simulink model "PMSM_U_F_PWM"  (R2020a)
settings: Solver=ode3  StartTime=0.0  StopTime=0.5  FixedStep=1e-5  RelTol=1e-3  EnableMultiTasking=on
model workspace (MAT data in the model file):
  B = 2.3e-05
  J = 6.5e-05
  KC = 0.04
  KV = 0.021
  L = 0.00021
  PP = 3
  Power_Supply_V = 18
  R = 0.215
  RLoad = 10
  T_FST_LP = 0.00012
undefined symbols (not defined in the file): sigbuilder_block
libraries: ammclib_bam x3, simulink x1
settings Model: Creator=admin_aboyer  LastModifiedBy=bourlot
settings DataIOCC: ExternalInput=off  InitialState=off  SaveOutput=off  SignalLogging=off  SaveTime=off  ReturnWorkspaceOutputs=off
settings OptimizationCC: BlockReduction=off  DefaultParameterBehavior=Inlined  LifeSpan=1  EfficientTunableParamExpr=on
settings DebuggingCC: InheritedTsInSrcMsg=none  MultiTaskDSMMsg=none  MultiTaskRateTransMsg=warning  SingleTaskRateTransMsg=warning  UnconnectedInputMsg=error  UnconnectedOutputMsg=error  UnconnectedLineMsg=error  UnknownTsInhSupMsg=error  SFUnexpectedBacktrackingDiag=warning  SFNoUnconditionalDefaultTransitionDiag=warning  ArithmeticOperatorsInVariantConditions=warning
settings HardwareCC: ProdBitPerPointer=32  ProdBitPerSizeT=32  ProdBitPerPtrDiffT=32  ProdLargestAtomicInteger=Long  ProdLargestAtomicFloat=Double  ProdEndianess=BigEndian  ProdWordSize=32  ProdHWDeviceType=Motorola PowerPC
settings SFSimCC: SimUseLocalCustomCode=off  MATLABDynamicMemAlloc=off  CustomCodeUndefinedFunction=UseInterfaceOnly
settings RTWCC: Description=Model Based Design Toolbox MPC574xP Code Generation Target  SystemTargetFile=mbd_pnt.tlc  MakeCommand=mbd_pnt_make_rtw COPY_MDLREF_INCLUDES=0  TemplateMakefile=mbd_pnt.tmf  GenerateReport=on  RTWUseLocalCustomCode=off  IncludeHyperlinkInReport=on  LaunchReport=on  GenerateTraceInfo=on  GenerateTraceReport=on  GenerateTraceReportSl=on  GenerateTraceReportSf=on  GenerateTraceReportEml=on
settings CodeAppCC: ForceParamTrailComments=on  IgnoreCustomStorageClasses=off  OperatorAnnotations=on  SimulinkDataObjDesc=on  SFDataObjDesc=on  MATLABFcnDesc=on  InsertBlockDesc=on  StateflowObjectComments=on  MATLABSourceComments=on
settings STFCustomTargetCC: GenerateSampleERTMain=on  CombineOutputUpdateFcns=on  SuppressErrorStatus=on  ERTCustomFileBanners=on  SupportContinuousTime=off  SupportNonInlinedSFcns=off  RemoveResetFunc=on  MATLABClassNameForMDSCustomization=Simulink.SoftwareTarget.ERTCustomization  SystemTargetFile=mbd_pnt.tlc
settings ERTTargetCC: MultiwordLength=2048  GenerateSampleERTMain=on  ParMdlRefBuildCompliant=off  CompOptLevelCompliant=off  ConcurrentExecutionCompliant=off  SuppressErrorStatus=on  ModelStepFunctionPrototypeControlCompliant=off  CPPClassGenCompliant=off  UseToolchainInfoCompliant=off  InlinedParameterPlacement=NonHierarchical  ERTCustomFileTemplate=example_file_process.tlc
settings ConfigComp: CovMetricSettings=dw  CovHtmlReporting=on  CovSaveCumulativeToWorkspaceVar=on  CovSaveSingleToWorkspaceVar=on  CovExternalEMLEnable=off

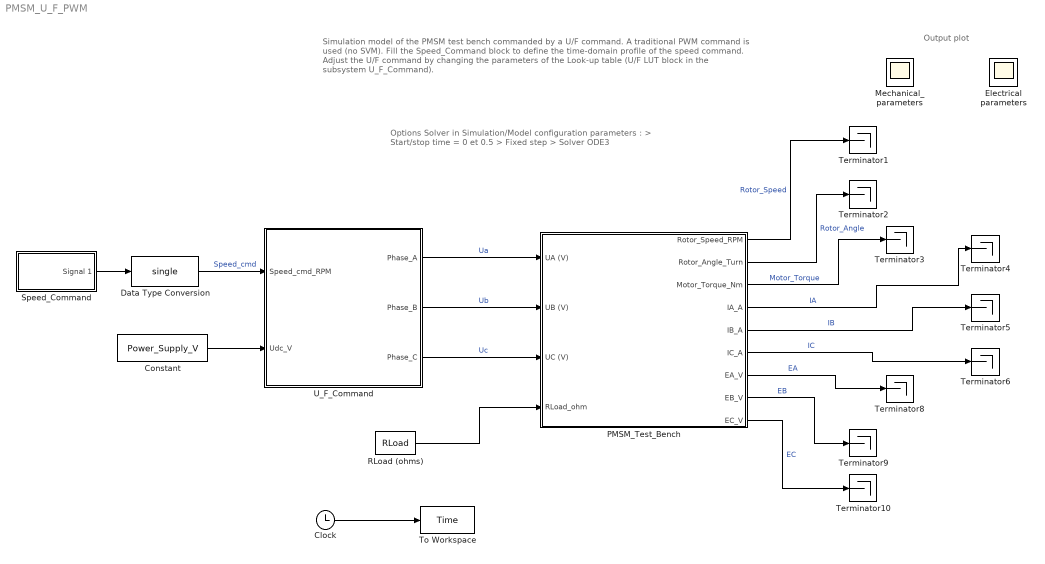
== system PMSM_U_F_PWM ==
  note: Output plot
  note: Options Solver in Simulation/Model configuration parameters :
      | >  Start/stop time = 0 et 0.5
      | >  Fixed step
      | >  Solver ODE3
  note: Simulation model of the PMSM test bench commanded by a U/F command.
      | A traditional PWM command is used (no SVM).
      | Fill the Speed_Command block to define the time-domain profile of the speed command.
      | Adjust the U/F command by changing the parameters of the Look-up table (U/F LUT
      | block in the subsystem U_F_Command).
  Clock : Clock
  Constant : Constant  Value=Power_Supply_V  OutDataTypeStr=single
  Data Type Conversion : DataTypeConversion  OutDataTypeStr=single
  Electrical parameters : Scope
      settings: Floating=on
  Mechanical_parameters : Scope
      settings: Floating=on
  PMSM_Test_Bench : Subsystem
  RLoad (ohms) : Constant  Value=RLoad
  Speed_Command : Subsystem  Tag=STV Subsys  LoadFcn=sigbuilder_block('load');  StartFcn=sigbuilder_block('start');  StopFcn=sigbuilder_block('stop');  ClipboardFcn=sigbuilder_block('clipboard');  mask(Sigbuilder block){tuvar=[0:10]}
      mask help: Simulink:masks:SigbuilderBlock_MD
      mask init:
      | if ~strcmp(get_param(bdroot(gcbh),'SimulationStatus'),'stopped') tuvar = sigbuilder_block('maskInit'); end
      settings: CopyFcn=sigbuilder_block('copy');  DeleteFcn=sigbuilder_block('delete');  ModelCloseFcn=sigbuilder_block('modelClose');  PreSaveFcn=sigbuilder_block('preSave');  PauseFcn=sigbuilder_block('pause');  ContinueFcn=sigbuilder_block('continue');  NameChangeFcn=sigbuilder_block('namechange');  OpenFcn=sigbuilder_block('open',[437.25 153.75 550.5 359.25 ]);  CloseFcn=sigbuilder_block('close');
      mask Display: plot(0, 0, 100, 100,[2, 2, 32, 32, 2], [68, 8, 8, 68, 68],[32, 2], [38, 38], [32, 19, 2],[53, 60, 44], [32, 17, 17, 2],[16, 16, 31, 31]);txt = getActiveGroup(gcbh);text(2, 100, txt,'verticalAlignment', 'top');
  Terminator{1..6,8..10} (9 alike) : Terminator
  To Workspace : ToWorkspace  VariableName=Time  SampleTime=-1
  U_F_Command : Subsystem
  wires:
  Clock/1 -> To Workspace/1
  U_F_Command/1(Phase_A) -> PMSM_Test_Bench/1(UA (V))  "Ua"
  U_F_Command/2(Phase_B) -> PMSM_Test_Bench/2(UB (V))  "Ub"
  U_F_Command/3(Phase_C) -> PMSM_Test_Bench/3(UC (V))  "Uc"
  PMSM_Test_Bench/1(Rotor_Speed_RPM) -> Terminator1/1  "Rotor_Speed"
  PMSM_Test_Bench/2(Rotor_Angle_Turn) -> Terminator2/1  "Rotor_Angle"
  PMSM_Test_Bench/3(Motor_Torque_Nm) -> Terminator3/1  "Motor_Torque"
  PMSM_Test_Bench/4(IA_A) -> Terminator4/1  "IA"
  PMSM_Test_Bench/5(IB_A) -> Terminator5/1  "IB"
  PMSM_Test_Bench/6(IC_A) -> Terminator6/1  "IC"
  PMSM_Test_Bench/7(EA_V) -> Terminator8/1  "EA"
  PMSM_Test_Bench/8(EB_V) -> Terminator9/1  "EB"
  PMSM_Test_Bench/9(EC_V) -> Terminator10/1  "EC"
  RLoad (ohms)/1 -> PMSM_Test_Bench/4(RLoad_ohm)
  Speed_Command/1(Signal 1) -> Data Type Conversion/1
  Data Type Conversion/1 -> U_F_Command/1(Speed_cmd_RPM)  "Speed_cmd"
  Constant/1 -> U_F_Command/2(Udc_V)

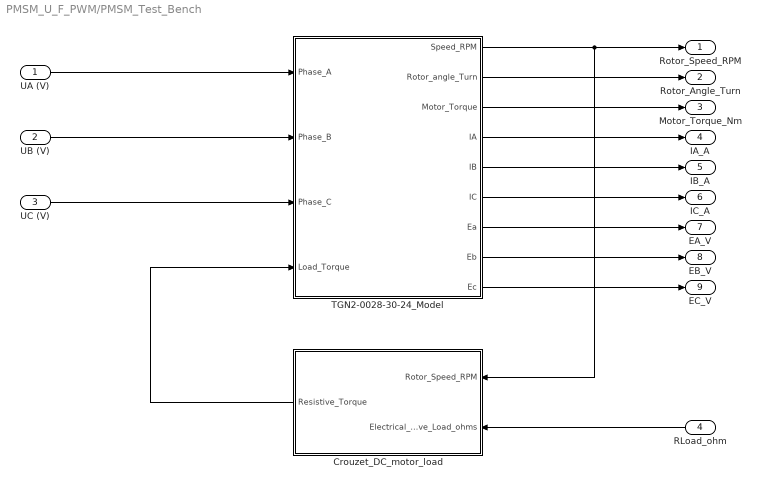
== system PMSM_U_F_PWM/PMSM_Test_Bench ==
  UA (V) : Inport
  UB (V) : Inport  Port=2
  UC (V) : Inport  Port=3
  RLoad_ohm : Inport  Port=4
  Crouzet_DC_motor_load : Subsystem
  TGN2-0028-30-24_Model : Subsystem
      mask Display: image('C:\WORKSPACE_MATLAB\PMSM_Workshop\M5\img\PMSM.PNG');
  Rotor_Speed_RPM : Outport
  Rotor_Angle_Turn : Outport  Port=2
  Motor_Torque_Nm : Outport  Port=3
  IA_A : Outport  Port=4
  IB_A : Outport  Port=5
  IC_A : Outport  Port=6
  EA_V : Outport  Port=7
  EB_V : Outport  Port=8
  EC_V : Outport  Port=9
  wires:
  Crouzet_DC_motor_load/1(Resistive_Torque) -> TGN2-0028-30-24_Model/4(Load_Torque)
  TGN2-0028-30-24_Model/1(Speed_RPM) -> Rotor_Speed_RPM/1, Crouzet_DC_motor_load/1(Rotor_Speed_RPM)
  UA (V)/1 -> TGN2-0028-30-24_Model/1(Phase_A)
  UB (V)/1 -> TGN2-0028-30-24_Model/2(Phase_B)
  UC (V)/1 -> TGN2-0028-30-24_Model/3(Phase_C)
  TGN2-0028-30-24_Model/2(Rotor_angle_Turn) -> Rotor_Angle_Turn/1
  TGN2-0028-30-24_Model/3(Motor_Torque) -> Motor_Torque_Nm/1
  TGN2-0028-30-24_Model/4(IA) -> IA_A/1
  TGN2-0028-30-24_Model/5(IB) -> IB_A/1
  TGN2-0028-30-24_Model/6(IC) -> IC_A/1
  TGN2-0028-30-24_Model/7(Ea) -> EA_V/1
  TGN2-0028-30-24_Model/8(Eb) -> EB_V/1
  TGN2-0028-30-24_Model/9(Ec) -> EC_V/1
  RLoad_ohm/1 -> Crouzet_DC_motor_load/2(Electrical_resistive_Load_ohms)

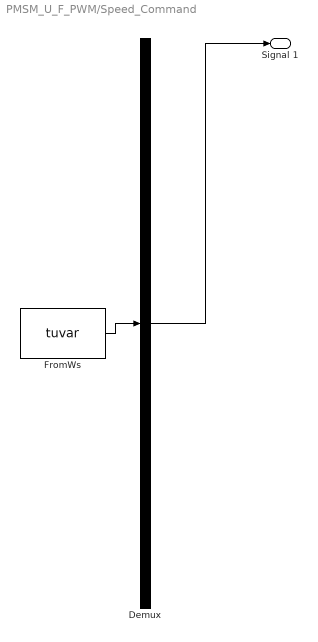
== system PMSM_U_F_PWM/Speed_Command ==
  Demux : Demux  Tag=STV Demux  Outputs=1
      settings: DisplayOption=none
  FromWs : FromWorkspace  Tag=STV FromWs  VariableName=tuvar
      SigBuilderData=|
      | common.afterFinalStr = 'Extrapolate'
      | common.sampleTime = 0
      | dataSet.timeRange = [0 10]
      | dataSet.name = 'Group 1'
      | sbobj.Groups.Name = 'Group 1'
      | sbobj.Groups.Signals.Name = 'Signal 1'
      | sbobj.Groups.Signals.XData = [0 0.2 6 10]
      | sbobj.Groups.Signals.YData = [0 1000 1000 0]
  Signal 1 : Outport  Tag=STV Outport
  wires:
  Demux/1 -> Signal 1/1
  FromWs/1 -> Demux/1

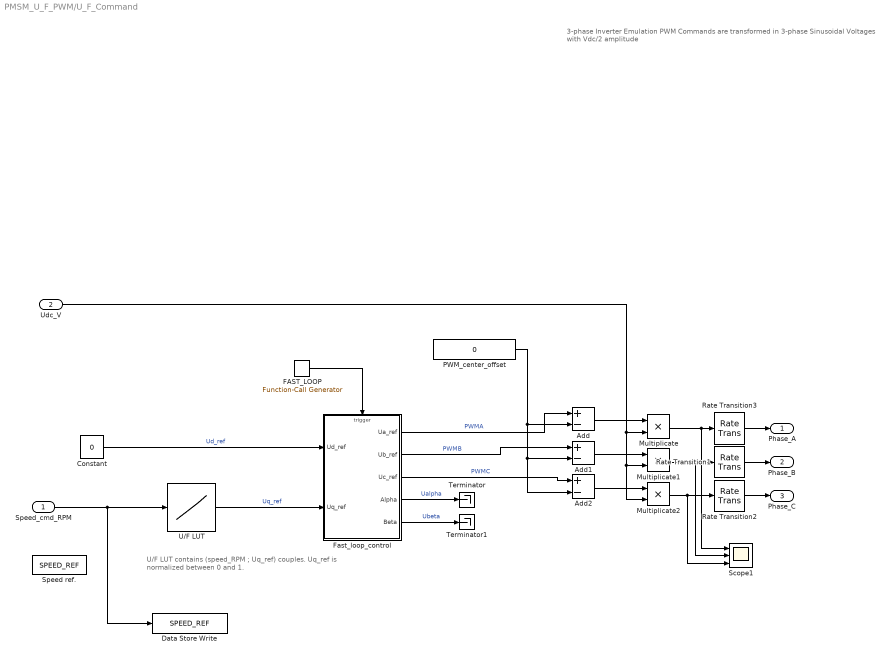
== system PMSM_U_F_PWM/U_F_Command ==
  note: U/F LUT contains (speed_RPM ; Uq_ref) couples. Uq_ref
      | is normalized between 0 and 1.
  note: 3-phase Inverter Emulation
      |
      | PWM Commands are transformed in 3-phase Sinusoidal Voltages with Vdc/2 amplitude
  Speed_cmd_RPM : Inport  OutDataTypeStr=single
  Udc_V : Inport  Port=2
  Add : Sum  Inputs=+-  OutDataTypeStr=single
  Add1 : Sum  Inputs=+-  OutDataTypeStr=single
  Add2 : Sum  Inputs=+-  OutDataTypeStr=single
  Constant : Constant  Value=0  OutDataTypeStr=single
  Data Store Write : DataStoreWrite  DataStoreName=SPEED_REF
  FAST_LOOP : simulink/Ports & Subsystems/Function-Call Generator  sample_time=T_FST_LP  numberOfIterations=1
  Fast_loop_control : Subsystem
  Multiplicate : Product  Inputs=**  OutDataTypeStr=single
  Multiplicate1 : Product  Inputs=**  OutDataTypeStr=single
  Multiplicate2 : Product  Inputs=**  OutDataTypeStr=single
  PWM_center_offset : Constant  Value=0  OutDataTypeStr=single
  Rate Transition1 : RateTransition
  Rate Transition2 : RateTransition
  Rate Transition3 : RateTransition
  Scope1 : Scope  NumInputPorts=3
  Speed ref. : DataStoreMemory  DataStoreName=SPEED_REF  ReadBeforeWriteMsg=warning  WriteAfterWriteMsg=warning  WriteAfterReadMsg=warning  ShowAdditionalParam=off  OutDataTypeStr=single
  Terminator : Terminator
  Terminator1 : Terminator
  U/F LUT : Lookup_n-D  NumberOfTableDimensions=1  BreakpointsForDimension1=[0,500,1000,2571,3000]  Table=[0.194,0.194,0.39,1,1]  InternalRulePriority=Speed  RndMeth=Simplest  InputSameDT=on
  Phase_A : Outport
  Phase_B : Outport  Port=2
  Phase_C : Outport  Port=3
  wires:
  FAST_LOOP/1 -> Fast_loop_control/Trigger
  Fast_loop_control/1(Ua_ref) -> Add/1  "PWMA"
  Fast_loop_control/2(Ub_ref) -> Add1/1  "PWMB"
  Fast_loop_control/3(Uc_ref) -> Add2/1  "PWMC"
  Speed_cmd_RPM/1 -> U/F LUT/1, Data Store Write/1
  Constant/1 -> Fast_loop_control/1(Ud_ref)  "Ud_ref"
  Fast_loop_control/4(Alpha) -> Terminator/1  "Ualpha"
  Fast_loop_control/5(Beta) -> Terminator1/1  "Ubeta"
  U/F LUT/1 -> Fast_loop_control/2(Uq_ref)  "Uq_ref"
  PWM_center_offset/1 -> Add/2, Add1/2, Add2/2
  Add/1 -> Multiplicate/1
  Multiplicate/1 -> Scope1/1, Rate Transition3/1
  Add1/1 -> Multiplicate1/1
  Add2/1 -> Multiplicate2/1
  Multiplicate1/1 -> Scope1/2, Rate Transition1/1
  Multiplicate2/1 -> Scope1/3, Rate Transition2/1
  Rate Transition3/1 -> Phase_A/1
  Rate Transition1/1 -> Phase_B/1
  Rate Transition2/1 -> Phase_C/1
  Udc_V/1 -> Multiplicate2/2, Multiplicate1/2, Multiplicate/2

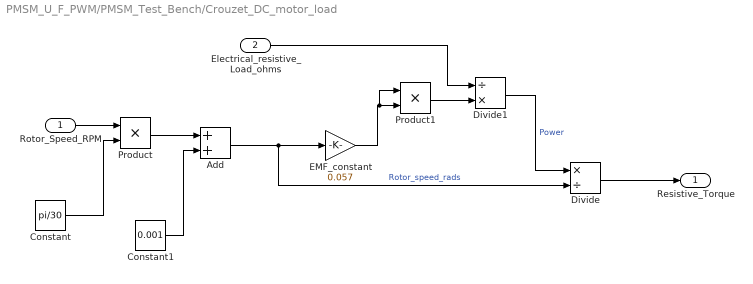
== system PMSM_U_F_PWM/PMSM_Test_Bench/Crouzet_DC_motor_load ==
  Rotor_Speed_RPM : Inport
  Electrical_resistive_Load_ohms : Inport  Port=2
  Add : Sum
  Constant : Constant  Value=pi/30
  Constant1 : Constant  Value=0.001
  Divide : Product  Inputs=*/
  Divide1 : Product  Inputs=/*
  EMF_constant : Gain  Gain=0.057
  Product : Product
  Product1 : Product
  Resistive_Torque : Outport
  wires:
  Rotor_Speed_RPM/1 -> Product/1
  Constant/1 -> Product/2
  Product/1 -> Add/1
  Constant1/1 -> Add/2
  Add/1 -> Divide/2, EMF_constant/1  "Rotor_speed_rads"
  EMF_constant/1 -> Product1/1, Product1/2
  Product1/1 -> Divide1/2
  Divide1/1 -> Divide/1  "Power"
  Divide/1 -> Resistive_Torque/1
  Electrical_resistive_Load_ohms/1 -> Divide1/1

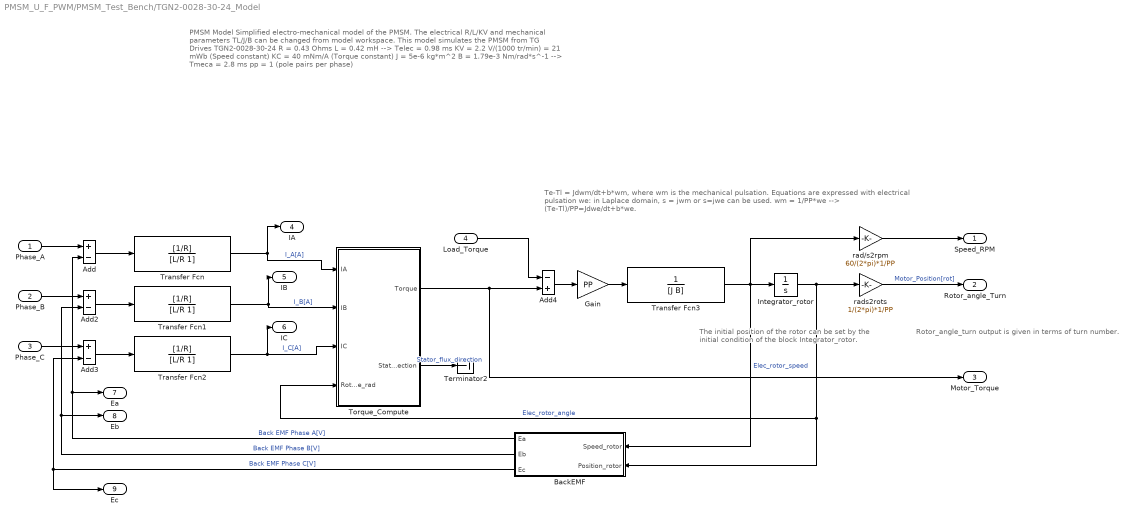
== system PMSM_U_F_PWM/PMSM_Test_Bench/TGN2-0028-30-24_Model ==
  note: The initial position of the rotor can be set by the
      | initial condition of the block Integrator_rotor.
  note: Te-Tl = Jdwm/dt+b*wm, where wm is the mechanical pulsation.
      | Equations are expressed with electrical pulsation we: in Laplace domain, s = jwm or s=jwe can be used.
      | wm = 1/PP*we --> (Te-Tl)/PP=Jdwe/dt+b*we.
  note: PMSM Model
      |
      | Simplified electro-mechanical model of the PMSM. The electrical R/L/KV and mechanical parameters TL/J/B can be changed from model workspace.
      |
      | This model simulates the PMSM from TG Drives TGN2-0028-30-24
      | R = 0.43 Ohms
      | L = 0.42 mH --> Telec = 0.98 ms
      | KV = 2.2 V/(1000 tr/min) = 21 mWb (Speed constant)
      | KC = 40 mNm/A (Torque constant)
      | J = 5e-6 kg*m^2
      | B = 1.79e-3 Nm/rad*s^-1 --> Tmeca = 2.8 ms
      | pp = 1 (pole pairs per phase)
  note: Rotor_angle_turn output is given in terms of turn number.
  Phase_A : Inport
  Phase_B : Inport  Port=2
  Phase_C : Inport  Port=3
  Load_Torque : Inport  Port=4
  Add : Sum  Inputs=+-
  Add2 : Sum  Inputs=+-
  Add3 : Sum  Inputs=+-
  Add4 : Sum  Inputs=-+
  BackEMF : Subsystem
  Gain : Gain  Gain=PP
  Integrator_rotor : Integrator  InitialCondition=-pi/2
  Terminator2 : Terminator
  Torque_Compute : Subsystem
  Transfer Fcn : TransferFcn  Numerator=[1/R]  Denominator=[L/R 1]
  Transfer Fcn1 : TransferFcn  Numerator=[1/R]  Denominator=[L/R 1]
  Transfer Fcn2 : TransferFcn  Numerator=[1/R]  Denominator=[L/R 1]
  Transfer Fcn3 : TransferFcn  Denominator=[J B]
  rad/s2rpm : Gain  Gain=60/(2*pi)*1/PP
  rads2rots : Gain  Gain=1/(2*pi)*1/PP
  Speed_RPM : Outport
  Rotor_angle_Turn : Outport  Port=2
  Motor_Torque : Outport  Port=3
  IA : Outport  Port=4
  IB : Outport  Port=5
  IC : Outport  Port=6
  Ea : Outport  Port=7
  Eb : Outport  Port=8
  Ec : Outport  Port=9
  wires:
  Add/1 -> Transfer Fcn/1
  Phase_A/1 -> Add/1
  Transfer Fcn/1 -> Torque_Compute/1(IA), IA/1  "I_A[A]"
  Transfer Fcn1/1 -> IB/1, Torque_Compute/2(IB)  "I_B[A]"
  Add2/1 -> Transfer Fcn1/1
  Add3/1 -> Transfer Fcn2/1
  Transfer Fcn2/1 -> IC/1, Torque_Compute/3(IC)  "I_C[A]"
  Phase_B/1 -> Add2/1
  Phase_C/1 -> Add3/1
  Load_Torque/1 -> Add4/1
  Add4/1 -> Gain/1
  Gain/1 -> Transfer Fcn3/1
  Transfer Fcn3/1 -> BackEMF/1(Speed_rotor), Integrator_rotor/1, rad/s2rpm/1  "Elec_rotor_speed"
  Torque_Compute/1(Torque) -> Motor_Torque/1, Add4/2
  BackEMF/3(Ec) -> Add3/2, Ec/1  "Back EMF Phase C[V]"
  BackEMF/1(Ea) -> Ea/1, Add/2  "Back EMF Phase A[V]"
  BackEMF/2(Eb) -> Eb/1, Add2/2  "Back EMF Phase B[V]"
  rad/s2rpm/1 -> Speed_RPM/1
  Integrator_rotor/1 -> Torque_Compute/4(Rotor_angle_rad), BackEMF/2(Position_rotor), rads2rots/1  "Elec_rotor_angle"
  rads2rots/1 -> Rotor_angle_Turn/1  "Motor_Position[rot]"
  Torque_Compute/2(Stator_Flux_Direction) -> Terminator2/1  "Stator_flux_direction"

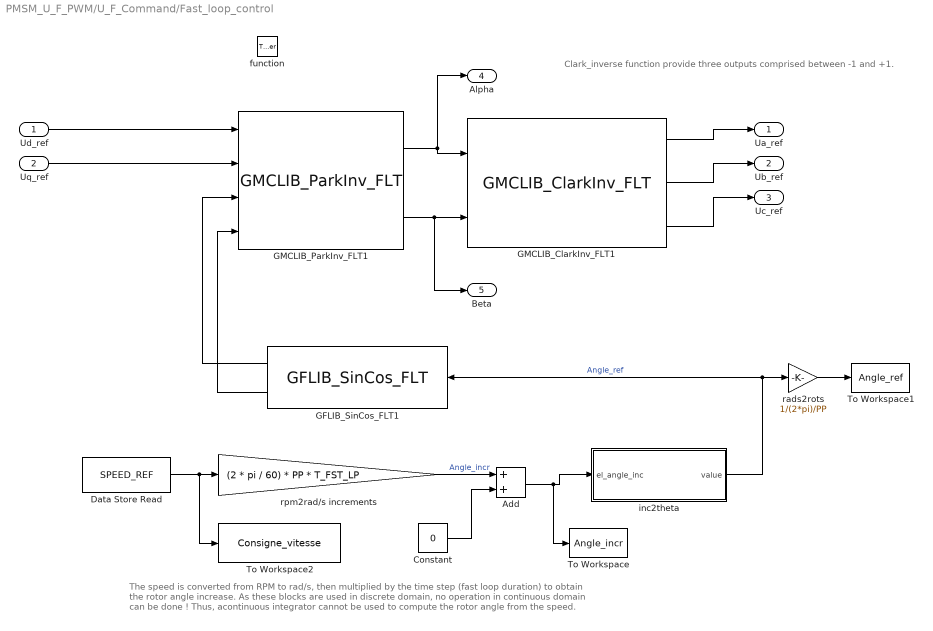
== system PMSM_U_F_PWM/U_F_Command/Fast_loop_control ==
  note: Clark_inverse function provide three outputs comprised between -1 and +1.
  note: The speed is converted from RPM to rad/s, then multiplied by the time step (fast loop duration) to obtain the rotor angle increase.
      | As these blocks are used in discrete domain, no operation in continuous domain can be done ! Thus, acontinuous integrator
      | cannot be used to compute the rotor angle from the speed.
  Ud_ref : Inport
  Uq_ref : Inport  Port=2
  function : TriggerPort  TriggerType=function-call  VariantControl=Variant
  Add : Sum
  Constant : Constant  Value=0  OutDataTypeStr=single
  Data Store Read : DataStoreRead  DataStoreName=SPEED_REF
  GFLIB_SinCos_FLT1 : ammclib_bam/GFLIB/FLT/GFLIB_SinCos_FLT
  GMCLIB_ClarkInv_FLT1 : ammclib_bam/GMCLIB/FLT/GMCLIB_ClarkInv_FLT
  GMCLIB_ParkInv_FLT1 : ammclib_bam/GMCLIB/FLT/GMCLIB_ParkInv_FLT
  To Workspace : ToWorkspace  VariableName=Angle_incr  SampleTime=-1
  To Workspace1 : ToWorkspace  VariableName=Angle_ref  SampleTime=-1
  To Workspace2 : ToWorkspace  VariableName=Consigne_vitesse  SampleTime=-1
  inc2theta : Stateflow chart  TreatAsAtomicUnit=on
      settings: RTWSystemCode=Nonreusable function  RTWFcnNameOpts=Use subsystem name
  rads2rots : Gain  Gain=1/(2*pi)/PP
  rpm2rad/s increments : Gain  Gain=(2 * pi / 60) * PP * T_FST_LP  OutDataTypeStr=single
  Ua_ref : Outport
  Ub_ref : Outport  Port=2
  Uc_ref : Outport  Port=3
  Alpha : Outport  Port=4
  Beta : Outport  Port=5
  wires:
  Data Store Read/1 -> To Workspace2/1, rpm2rad/s increments/1
  inc2theta/1(value) -> GFLIB_SinCos_FLT1/1, rads2rots/1  "Angle_ref"
  GFLIB_SinCos_FLT1/1 -> GMCLIB_ParkInv_FLT1/3
  GMCLIB_ParkInv_FLT1/1 -> GMCLIB_ClarkInv_FLT1/1, Alpha/1
  GMCLIB_ParkInv_FLT1/2 -> GMCLIB_ClarkInv_FLT1/2, Beta/1
  GMCLIB_ClarkInv_FLT1/3 -> Uc_ref/1
  GMCLIB_ClarkInv_FLT1/2 -> Ub_ref/1
  GMCLIB_ClarkInv_FLT1/1 -> Ua_ref/1
  rads2rots/1 -> To Workspace1/1
  rpm2rad/s increments/1 -> Add/1  "Angle_incr"
  Add/1 -> To Workspace/1, inc2theta/1(el_angle_inc)
  Constant/1 -> Add/2
  Uq_ref/1 -> GMCLIB_ParkInv_FLT1/2
  Ud_ref/1 -> GMCLIB_ParkInv_FLT1/1
  GFLIB_SinCos_FLT1/2 -> GMCLIB_ParkInv_FLT1/4

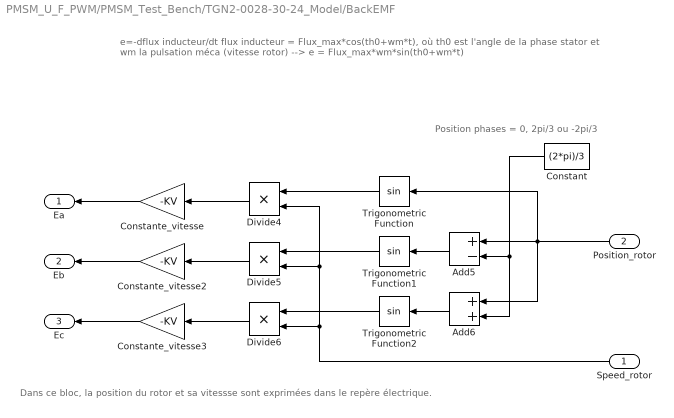
== system PMSM_U_F_PWM/PMSM_Test_Bench/TGN2-0028-30-24_Model/BackEMF ==
  note: Dans ce bloc, la position du rotor et sa vitessse sont exprimées dans le repère électrique.
  note: e=-dflux inducteur/dt
      | flux inducteur = Flux_max*cos(th0+wm*t), où th0 est l'angle de la phase stator et wm la pulsation méca (vitesse rotor)
      | --> e = Flux_max*wm*sin(th0+wm*t)
  note: Position phases = 0, 2pi/3 ou -2pi/3
  Speed_rotor : Inport
  Position_rotor : Inport  Port=2
  Add5 : Sum  Inputs=+-
  Add6 : Sum
  Constant : Constant  Value=(2*pi)/3
  Constante_vitesse : Gain  Gain=-KV
  Constante_vitesse2 : Gain  Gain=-KV
  Constante_vitesse3 : Gain  Gain=-KV
  Divide4 : Product  Inputs=**
  Divide5 : Product  Inputs=**
  Divide6 : Product  Inputs=**
  Trigonometric Function : Trigonometry
  Trigonometric Function1 : Trigonometry
  Trigonometric Function2 : Trigonometry
  Ea : Outport
  Eb : Outport  Port=2
  Ec : Outport  Port=3
  wires:
  Divide4/1 -> Constante_vitesse/1
  Divide6/1 -> Constante_vitesse3/1
  Trigonometric Function2/1 -> Divide6/1
  Constante_vitesse3/1 -> Ec/1
  Speed_rotor/1 -> Divide4/2, Divide5/2, Divide6/2
  Constante_vitesse2/1 -> Eb/1
  Divide5/1 -> Constante_vitesse2/1
  Constant/1 -> Add6/2, Add5/2
  Add6/1 -> Trigonometric Function2/1
  Trigonometric Function/1 -> Divide4/1
  Add5/1 -> Trigonometric Function1/1
  Constante_vitesse/1 -> Ea/1
  Trigonometric Function1/1 -> Divide5/1
  Position_rotor/1 -> Add5/1, Trigonometric Function/1, Add6/1

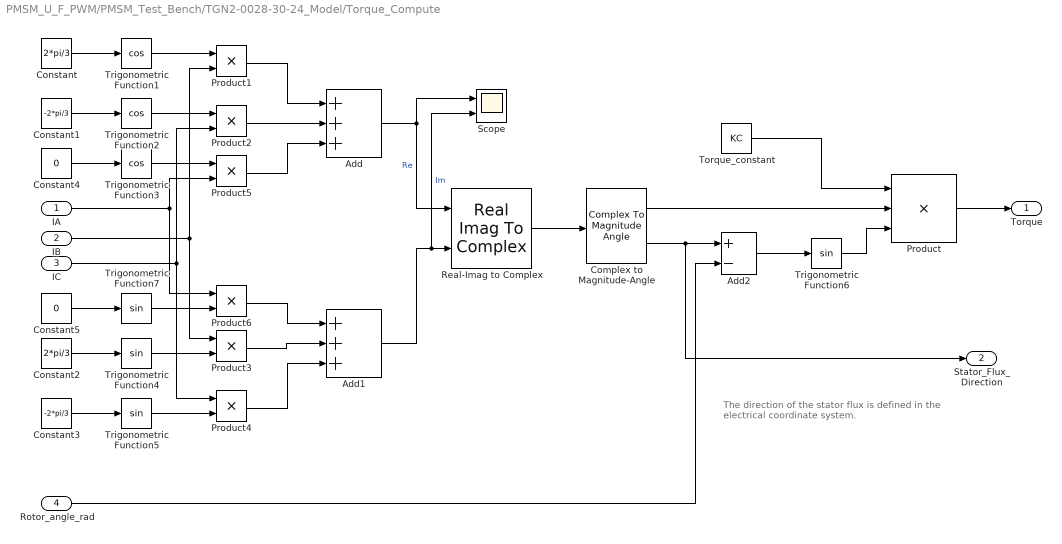
== system PMSM_U_F_PWM/PMSM_Test_Bench/TGN2-0028-30-24_Model/Torque_Compute ==
  note: The direction of the stator flux is defined in the
      | electrical coordinate system.
  IA : Inport
  IB : Inport  Port=2
  IC : Inport  Port=3
  Rotor_angle_rad : Inport  Port=4
  Add : Sum  Inputs=+++
  Add1 : Sum  Inputs=+++
  Add2 : Sum  Inputs=+-
  Complex to Magnitude-Angle : ComplexToMagnitudeAngle
  Constant : Constant  Value=2*pi/3
  Constant1 : Constant  Value=-2*pi/3
  Constant2 : Constant  Value=2*pi/3
  Constant3 : Constant  Value=-2*pi/3
  Constant4 : Constant  Value=0
  Constant5 : Constant  Value=0
  Product : Product  Inputs=3
  Product{1..6} (6 alike) : Product
  Real-Imag to Complex : RealImagToComplex
  Scope : Scope  NumInputPorts=2
  Torque_constant : Constant  Value=KC
  Trigonometric Function1 : Trigonometry  Operator=cos
  Trigonometric Function2 : Trigonometry  Operator=cos
  Trigonometric Function3 : Trigonometry  Operator=cos
  Trigonometric Function{4..7} (4 alike) : Trigonometry
  Torque : Outport
  Stator_Flux_Direction : Outport  Port=2
  wires:
  Add/1 -> Real-Imag to Complex/1, Scope/1  "Re"
  Add1/1 -> Scope/2, Real-Imag to Complex/2  "Im"
  Real-Imag to Complex/1 -> Complex to Magnitude-Angle/1
  Complex to Magnitude-Angle/2 -> Stator_Flux_Direction/1, Add2/1
  Rotor_angle_rad/1 -> Add2/2
  Add2/1 -> Trigonometric Function6/1
  Complex to Magnitude-Angle/1 -> Product/2
  Trigonometric Function6/1 -> Product/3
  Torque_constant/1 -> Product/1
  Product/1 -> Torque/1
  Constant1/1 -> Trigonometric Function2/1
  Constant/1 -> Trigonometric Function1/1
  Trigonometric Function1/1 -> Product1/1
  Trigonometric Function2/1 -> Product2/1
  IB/1 -> Product1/2, Product3/1
  IC/1 -> Product4/1, Product2/2
  Product1/1 -> Add/1
  Product2/1 -> Add/2
  Constant3/1 -> Trigonometric Function5/1
  Constant2/1 -> Trigonometric Function4/1
  Trigonometric Function4/1 -> Product3/2
  Trigonometric Function5/1 -> Product4/2
  Product3/1 -> Add1/2
  Product4/1 -> Add1/3
  Constant4/1 -> Trigonometric Function3/1
  Trigonometric Function3/1 -> Product5/1
  IA/1 -> Product6/1, Product5/2
  Product5/1 -> Add/3
  Trigonometric Function7/1 -> Product6/2
  Constant5/1 -> Trigonometric Function7/1
  Product6/1 -> Add1/1

== stateflow chart PMSM_U_F_PWM/U_F_Command/Fast_loop_control/inc2theta ==
  settings: executeAtInitialization=1
  state A
    du:
    value = value+el_angle_inc;
    ex:
    value = -3.14159+el_angle_inc;
  (default) -> A : {value = 0;}
  A -> A : [value > 3.14159]
  data: value output single; el_angle_inc input single
